simulink model "proiect"  (R2023a)
settings: Solver=VariableStepAuto  StartTime=0.0  StopTime=2000  RelTol=1e-3
values from neighbouring files (symbols this model uses):
  A = 332.5    [initializare_model.m]
  C = 6.95    [initializare_model.m]
  ho = 17.38    [initializare_model.m]
  k = 0.033    [initializare_model.m]
  k11 = k2^2 + 4*(k - k3)*k1    (= 0.0881226)    [initializare_model.m]
  k12 = 8*(k - k3)    (= 0.2688)    [initializare_model.m]
  k13 = 2*(k - k3)    (= 0.0672)    [initializare_model.m]
  k2 = -0.015    [initializare_model.m]
  keta = 8e-5    (= 8e-05)    [initializare_model.m]
  qo = 13    [initializare_model.m]
  uss = uo + 0.5    (= 5.8)    [initializare_model.m]
settings Model: Creator=evely  LastModifiedBy=evely

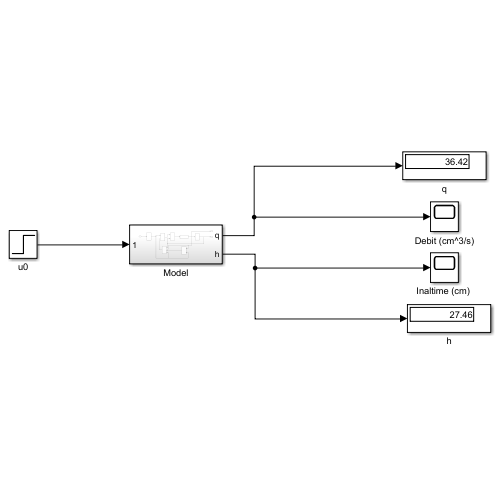
[thumbnail: Simulink's stored preview of the top-level diagram]
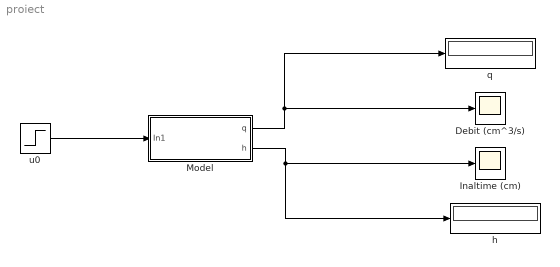
== system proiect ==
  Debit (cm^3/s) : Scope
  "Inaltime (cm) " : Scope
  Model : Subsystem
  h : Display
  q : Display
  u0 : Step  Time=0  After=uss  SampleTime=0
  wires:
  u0/1 -> Model/1(In1)
  Model/1(q) -> q/1, Debit (cm^3/s)/1
  Model/2(h) -> h/1, "Inaltime (cm) "/1

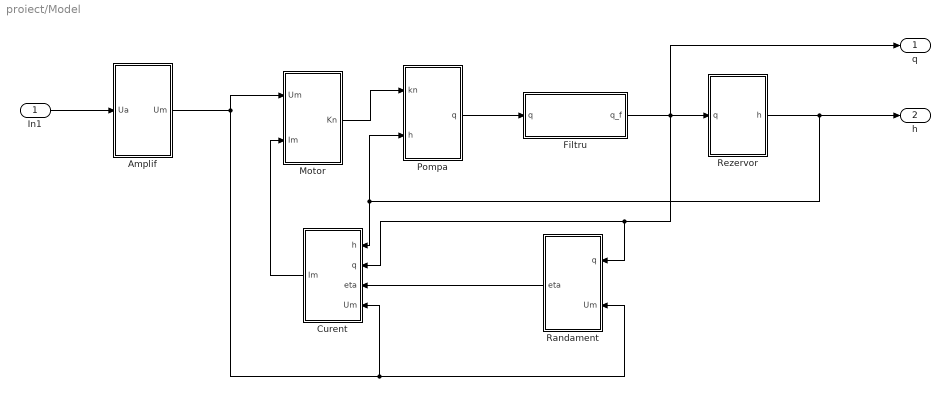
== system proiect/Model ==
  In1 : Inport
  Amplif : Subsystem
  Curent : Subsystem
  Filtru : Subsystem
  Motor : Subsystem
  Pompa : Subsystem
  Randament : Subsystem
  Rezervor : Subsystem
  q : Outport
  h : Outport  Port=2
  wires:
  In1/1 -> Amplif/1(Ua)
  Filtru/1(q_f) -> q/1, Randament/1(q), Curent/2(q), Rezervor/1(q)
  Rezervor/1(h) -> Pompa/2(h), Curent/1(h), h/1
  Amplif/1(Um) -> Motor/1(Um), Randament/2(Um), Curent/4(Um)
  Motor/1(Kn) -> Pompa/1(kn)
  Randament/1(eta) -> Curent/3(eta)
  Curent/1(Im) -> Motor/2(Im)
  Pompa/1(q) -> Filtru/1(q)

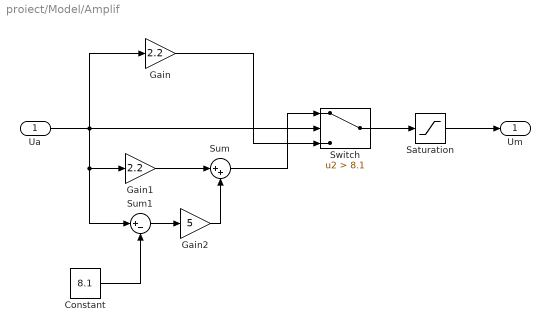
== system proiect/Model/Amplif ==
  Ua : Inport
  Constant : Constant  Value=8.1
  Gain : Gain  Gain=2.2
  Gain1 : Gain  Gain=2.2
  Gain2 : Gain  Gain=5
  Saturation : Saturate  UpperLimit=22  LowerLimit=0
  Sum : Sum  Inputs=|++
  Sum1 : Sum  Inputs=|+-
  Switch : Switch  Criteria=u2 > Threshold  Threshold=8.1  SaturateOnIntegerOverflow=off  InputSameDT=off
  Um : Outport
  wires:
  Ua/1 -> Gain1/1, Sum1/1, Gain/1, Switch/2
  Gain/1 -> Switch/3
  Switch/1 -> Saturation/1
  Gain1/1 -> Sum/1
  Constant/1 -> Sum1/2
  Sum1/1 -> Gain2/1
  Gain2/1 -> Sum/2
  Sum/1 -> Switch/1
  Saturation/1 -> Um/1

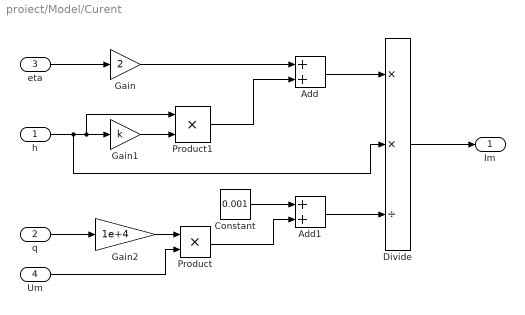
== system proiect/Model/Curent ==
  h : Inport
  q : Inport  Port=2
  eta : Inport  Port=3
  Um : Inport  Port=4
  Add : Sum
  Add1 : Sum
  Constant : Constant  Value=0.001
  Divide : Product  Inputs=**/
  Gain : Gain  Gain=2
  Gain1 : Gain  Gain=k
  Gain2 : Gain  Gain=1e+4
  Product : Product
  Product1 : Product
  Im : Outport
  wires:
  eta/1 -> Gain/1
  Gain/1 -> Add/1
  h/1 -> Divide/2, Product1/1, Gain1/1
  Gain1/1 -> Product1/2
  Add/1 -> Divide/1
  Product1/1 -> Add/2
  Divide/1 -> Im/1
  q/1 -> Gain2/1
  Gain2/1 -> Product/1
  Um/1 -> Product/2
  Constant/1 -> Add1/1
  Product/1 -> Add1/2
  Add1/1 -> Divide/3

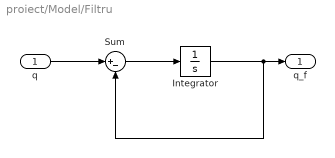
== system proiect/Model/Filtru ==
  q : Inport
  Integrator : Integrator  InitialCondition=qo
  Sum : Sum  Inputs=|+-
  q_f : Outport
  wires:
  q/1 -> Sum/1
  Sum/1 -> Integrator/1
  Integrator/1 -> Sum/2, q_f/1

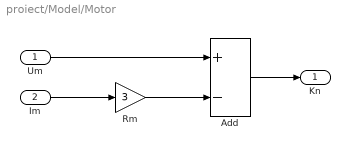
== system proiect/Model/Motor ==
  Um : Inport
  Im : Inport  Port=2
  Add : Sum  Inputs=+-
  Rm : Gain  Gain=3
  Kn : Outport
  wires:
  Im/1 -> Rm/1
  Rm/1 -> Add/2
  Um/1 -> Add/1
  Add/1 -> Kn/1

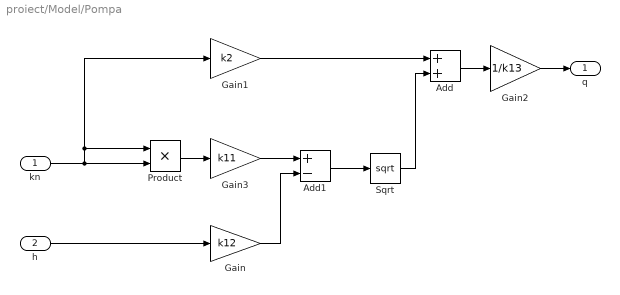
== system proiect/Model/Pompa ==
  kn : Inport
  h : Inport  Port=2
  Add : Sum
  Add1 : Sum  Inputs=+-
  Gain : Gain  Gain=k12
  Gain1 : Gain  Gain=k2
  Gain2 : Gain  Gain=1/k13
  Gain3 : Gain  Gain=k11
  Product : Product
  Sqrt : Sqrt
  q : Outport
  wires:
  kn/1 -> Product/1, Gain1/1, Product/2
  Gain1/1 -> Add/1
  Add/1 -> Gain2/1
  Gain2/1 -> q/1
  h/1 -> Gain/1
  Product/1 -> Gain3/1
  Gain3/1 -> Add1/1
  Add1/1 -> Sqrt/1
  Gain/1 -> Add1/2
  Sqrt/1 -> Add/2

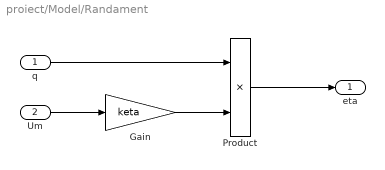
== system proiect/Model/Randament ==
  q : Inport
  Um : Inport  Port=2
  Gain : Gain  Gain=keta
  Product : Product
  eta : Outport
  wires:
  q/1 -> Product/1
  Product/1 -> eta/1
  Um/1 -> Gain/1
  Gain/1 -> Product/2

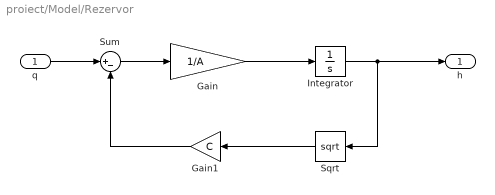
== system proiect/Model/Rezervor ==
  q : Inport
  Gain : Gain  Gain=1/A
  Gain1 : Gain  Gain=C
  Integrator : Integrator  InitialCondition=ho
  Sqrt : Sqrt
  Sum : Sum  Inputs=|+-
  h : Outport
  wires:
  q/1 -> Sum/1
  Sum/1 -> Gain/1
  Gain/1 -> Integrator/1
  Integrator/1 -> Sqrt/1, h/1
  Sqrt/1 -> Gain1/1
  Gain1/1 -> Sum/2
